simulink model "Essaie_01"  (R2021a)
settings: Solver=FixedStepDiscrete  StartTime=0.0  StopTime=8.75  RelTol=1e-3  EnableMultiTasking=on
libraries: simulink x8, simulink_extras x2, dspsigops x2, dsparch4 x2, commfilt2 x2
settings Model: Creator=sebastienroy  LastModifiedBy=Simon
settings SolverCC: AlgebraicLoopSolver=TrustRegion
settings DataIOCC: LimitDataPoints=on  SaveFormat=Array  ReturnWorkspaceOutputs=off
settings OptimizationCC: LifeSpan=inf
settings DebuggingCC: UnderspecifiedInitializationDetection=Classic  MergeDetectMultiDrivingBlocksExec=none  SolverPrmCheckMsg=warning  StateNameClashWarn=warning  SFUnexpectedBacktrackingDiag=warning  SFNoUnconditionalDefaultTransitionDiag=warning  SFExecutionAtInitializationDiag=none  SFMachineParentedDataDiag=warning  ArithmeticOperatorsInVariantConditions=warning
settings HardwareCC: ProdBitPerPointer=32  ProdBitPerSizeT=32  ProdBitPerPtrDiffT=32  ProdLargestAtomicFloat=None  ProdIntDivRoundTo=Undefined  ProdEndianess=Unspecified  ProdWordSize=32  ProdHWDeviceType=32-bit Generic
settings ModelReferenceCC: PropagateSignalLabelsOutOfModel=off
settings SFSimCC: SimUseLocalCustomCode=off  CustomCodeUndefinedFunction=UseInterfaceOnly
settings RTWCC: RTWUseLocalCustomCode=off
settings CodeAppCC: StateflowObjectComments=on
settings GRTTargetCC: TargetLangStandard=C89/C90 (ANSI)
settings ConfigComp: CovMetricSettings=dw  CovSaveCumulativeToWorkspaceVar=on  CovSaveSingleToWorkspaceVar=on  CovExternalEMLEnable=off

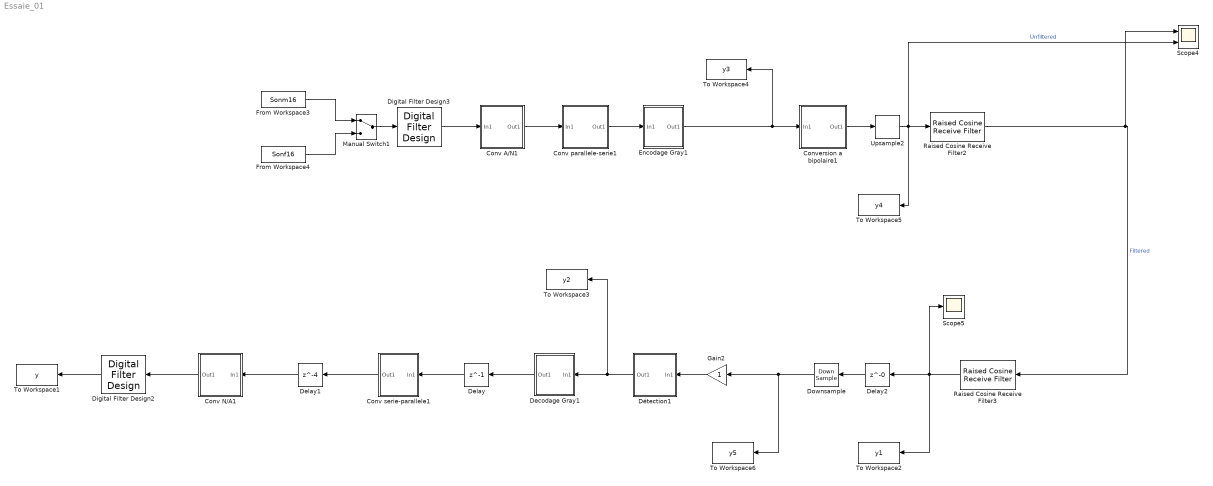
== system Essaie_01 ==
  Conv A/N1 : Subsystem
  Conv N/A1 : Subsystem
  Conv parallele-serie1 : Subsystem
  Conv serie-parallele1 : Subsystem
  Conversion a bipolaire1 : Subsystem
  Decodage Gray1 : Subsystem
  Delay : Delay  DelayLength=1  InitialCondition=0
  Delay1 : Delay  DelayLength=4  InitialCondition=0
  Delay2 : Delay  DelayLength=0  InitialCondition=0
  Digital Filter Design2 : dsparch4/Digital Filter Design  mwdsp_browser_bugfix_var=off
  Digital Filter Design3 : dsparch4/Digital Filter Design  mwdsp_browser_bugfix_var=off
  Downsample : DownSample  N=20  RateOptions=Allow multirate processing
  Détection1 : Subsystem
  Encodage Gray1 : Subsystem
  From Workspace3 : FromWorkspace  VariableName=Sonm16  SampleTime=1/16000  Interpolate=off  OutputAfterFinalValue=Setting to zero
  From Workspace4 : FromWorkspace  VariableName=Sonf16  SampleTime=1/16000  Interpolate=off  OutputAfterFinalValue=Setting to zero
  Gain2 : Gain
  Manual Switch1 : ManualSwitch
  Raised Cosine Receive Filter2 : commfilt2/Raised Cosine Receive Filter  filtType=Square root  R=0.2  filtSpan=10  N=20  downFactor=1  downOffset=0  filterGain=1  RateOptions=Allow multirate processing  framing=Mute  checkCoeff=on  variableName=rcRxFilt2  currentFiltSpan=10  D=5  inputOffset=0  sampMode=Mute  saveAsFlag=0  rateMode=Downsampling  checkGain=Normalized  launchFVT=on  roundingMode=Floor  overflowMode=off  coeffDataTypeStr=Inherit: Same word length as input  coeffMin=[]  coeffMax=[]  coeffLastDataTypeStr=Inherit: Same word length as input  accumDataTypeStr=Inherit: Same as product output  accumLastDataTypeStr=Inherit: Same as product output  outputDataTypeStr=Inherit: Same as accumulator  outputMin=[]  outputMax=[]  outputLastDataTypeStr=Inherit: Same as accumulator
  Raised Cosine Receive Filter3 : commfilt2/Raised Cosine Receive Filter  filtType=Square root  R=0.2  filtSpan=10  N=20  downFactor=1  downOffset=0  filterGain=1  RateOptions=Allow multirate processing  framing=Mute  checkCoeff=on  variableName=rcRxFilt3  currentFiltSpan=10  D=5  inputOffset=0  sampMode=Mute  saveAsFlag=0  rateMode=Downsampling  checkGain=Normalized  launchFVT=on  roundingMode=Floor  overflowMode=off  coeffDataTypeStr=Inherit: Same word length as input  coeffMin=[]  coeffMax=[]  coeffLastDataTypeStr=Inherit: Same word length as input  accumDataTypeStr=Inherit: Same as product output  accumLastDataTypeStr=Inherit: Same as product output  outputDataTypeStr=Inherit: Same as accumulator  outputMin=[]  outputMax=[]  outputLastDataTypeStr=Inherit: Same as accumulator
  Scope4 : Scope  NumInputPorts=2
  Scope5 : Scope
  To Workspace1 : ToWorkspace  VariableName=y  SampleTime=-1
      settings: Save2DSignal=2-D array (concatenate along first dimension)
  To Workspace2 : ToWorkspace  VariableName=y1  SampleTime=-1
      settings: Save2DSignal=2-D array (concatenate along first dimension)
  To Workspace3 : ToWorkspace  VariableName=y2  SampleTime=-1
      settings: Save2DSignal=2-D array (concatenate along first dimension)
  To Workspace4 : ToWorkspace  VariableName=y3  SampleTime=-1
      settings: Save2DSignal=2-D array (concatenate along first dimension)
  To Workspace5 : ToWorkspace  VariableName=y4  SampleTime=-1
      settings: Save2DSignal=2-D array (concatenate along first dimension)
  To Workspace6 : ToWorkspace  VariableName=y5  SampleTime=-1
      settings: Save2DSignal=2-D array (concatenate along first dimension)
  Upsample2 : dspsigops/Upsample  N=20  phase=0  RateOptions=Allow multirate processing  ic=0  mode=Unused parameter value
  wires:
  Upsample2/1 -> Scope4/2, Raised Cosine Receive Filter2/1, To Workspace5/1  "Unfiltered"
  Encodage Gray1/1(Out1) -> To Workspace4/1, Conversion a bipolaire1/1(In1)
  Conv A/N1/1(Out1) -> Conv parallele-serie1/1(In1)
  Decodage Gray1/1(Out1) -> Delay/1
  Digital Filter Design3/1 -> Conv A/N1/1(In1)
  Gain2/1 -> Détection1/1(In1)
  Delay2/1 -> Downsample/1
  Conv N/A1/1(Out1) -> Digital Filter Design2/1
  From Workspace3/1 -> Manual Switch1/1
  Détection1/1(Out1) -> To Workspace3/1, Decodage Gray1/1(In1)
  Conversion a bipolaire1/1(Out1) -> Upsample2/1
  Conv parallele-serie1/1(Out1) -> Encodage Gray1/1(In1)
  Manual Switch1/1 -> Digital Filter Design3/1
  Downsample/1 -> To Workspace6/1, Gain2/1
  Delay/1 -> Conv serie-parallele1/1(In1)
  Raised Cosine Receive Filter2/1 -> Raised Cosine Receive Filter3/1, Scope4/1  "Filtered"
  Digital Filter Design2/1 -> To Workspace1/1
  From Workspace4/1 -> Manual Switch1/2
  Raised Cosine Receive Filter3/1 -> Scope5/1, To Workspace2/1, Delay2/1
  Delay1/1 -> Conv N/A1/1(In1)
  Conv serie-parallele1/1(Out1) -> Delay1/1

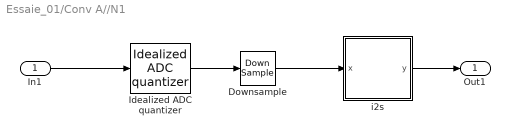
== system Essaie_01/Conv A//N1 ==
  In1 : Inport
  Downsample : DownSample  RateOptions=Allow multirate processing
  Idealized ADC quantizer : simulink_extras/Additional Discrete/Idealized ADC quantizer  NumberOfConverterBits=8  Vmin=-1  Vmax=1  OutputDataType=double  OutputNegativeValues=off
  i2s : Subsystem
  Out1 : Outport  VectorParamsAs1DForOutWhenUnconnected=off
  wires:
  Idealized ADC quantizer/1 -> Downsample/1
  In1/1 -> Idealized ADC quantizer/1
  Downsample/1 -> i2s/1(x)
  i2s/1(y) -> Out1/1

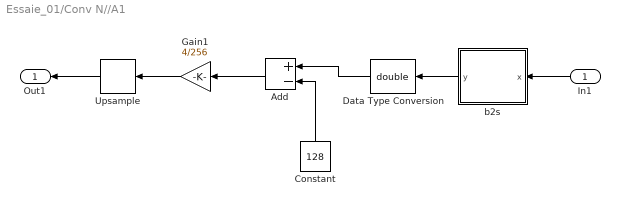
== system Essaie_01/Conv N//A1 ==
  In1 : Inport
  Add : Sum  Inputs=+-
  Constant : Constant  Value=128
  Data Type Conversion : DataTypeConversion  OutDataTypeStr=double
  Gain1 : Gain  Gain=4/256
  Upsample : dspsigops/Upsample  N=2  phase=0  RateOptions=Allow multirate processing  ic=0  mode=Unused parameter value
  b2s : Subsystem
  Out1 : Outport  VectorParamsAs1DForOutWhenUnconnected=off
  wires:
  Upsample/1 -> Out1/1
  Gain1/1 -> Upsample/1
  Constant/1 -> Add/2
  Data Type Conversion/1 -> Add/1
  Add/1 -> Gain1/1
  In1/1 -> b2s/1(x)
  b2s/1(y) -> Data Type Conversion/1

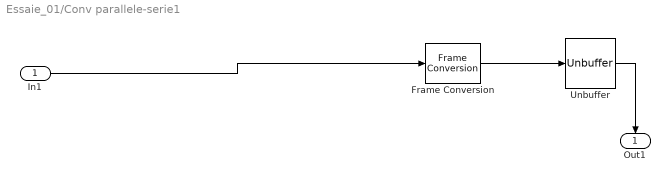
== system Essaie_01/Conv parallele-serie1 ==
  In1 : Inport
  Frame Conversion : FrameConversion
  Unbuffer : Unbuffer
  Out1 : Outport  VectorParamsAs1DForOutWhenUnconnected=off
  wires:
  Frame Conversion/1 -> Unbuffer/1
  Unbuffer/1 -> Out1/1
  In1/1 -> Frame Conversion/1

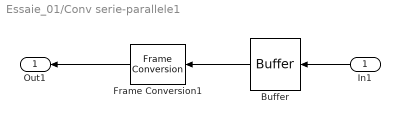
== system Essaie_01/Conv serie-parallele1 ==
  In1 : Inport
  Buffer : Buffer  N=4
  Frame Conversion1 : FrameConversion  OutFrame=Sample-based
  Out1 : Outport  VectorParamsAs1DForOutWhenUnconnected=off
  wires:
  Frame Conversion1/1 -> Out1/1
  In1/1 -> Buffer/1
  Buffer/1 -> Frame Conversion1/1

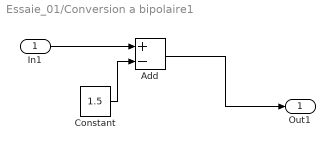
== system Essaie_01/Conversion a bipolaire1 ==
  In1 : Inport
  Add : Sum  Inputs=+-
  Constant : Constant  Value=1.5
  Out1 : Outport  VectorParamsAs1DForOutWhenUnconnected=off
  wires:
  In1/1 -> Add/1
  Add/1 -> Out1/1
  Constant/1 -> Add/2

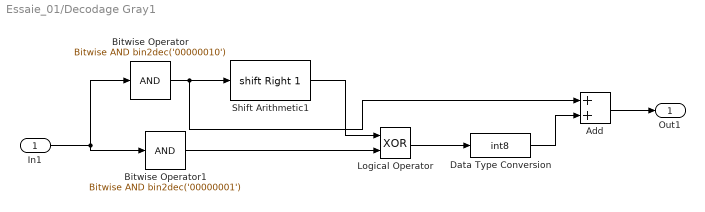
== system Essaie_01/Decodage Gray1 ==
  In1 : Inport
  Add : Sum
  Bitwise Operator : simulink/Logic and Bit Operations/Bitwise Operator  logicop=AND  UseBitMask=on  BitMask=bin2dec('00000010')  BitMaskRealWorld=Stored Integer
  Bitwise Operator1 : simulink/Logic and Bit Operations/Bitwise Operator  logicop=AND  UseBitMask=on  BitMask=bin2dec('00000001')  BitMaskRealWorld=Stored Integer
  Data Type Conversion : DataTypeConversion  OutDataTypeStr=int8
  Logical Operator : Logic  Operator=XOR  AllPortsSameDT=off
  Shift Arithmetic1 : ArithShift  BitShiftNumber=1  BitShiftDirection=Right
  Out1 : Outport  VectorParamsAs1DForOutWhenUnconnected=off
  wires:
  In1/1 -> Bitwise Operator/1, Bitwise Operator1/1
  Bitwise Operator/1 -> Add/1, Shift Arithmetic1/1
  Shift Arithmetic1/1 -> Logical Operator/1
  Bitwise Operator1/1 -> Logical Operator/2
  Add/1 -> Out1/1
  Logical Operator/1 -> Data Type Conversion/1
  Data Type Conversion/1 -> Add/2

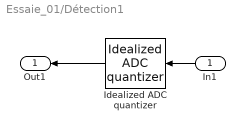
== system Essaie_01/Détection1 ==
  In1 : Inport
  Idealized ADC quantizer : simulink_extras/Additional Discrete/Idealized ADC quantizer  NumberOfConverterBits=2  Vmin=-1.5*20  Vmax=2.5*20  OutputDataType=int8  OutputNegativeValues=off
  Out1 : Outport
  wires:
  In1/1 -> Idealized ADC quantizer/1
  Idealized ADC quantizer/1 -> Out1/1

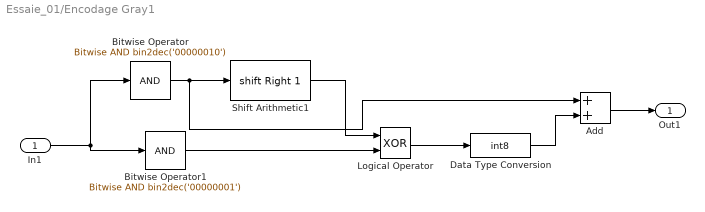
== system Essaie_01/Encodage Gray1 ==
  In1 : Inport
  Add : Sum
  Bitwise Operator : simulink/Logic and Bit Operations/Bitwise Operator  logicop=AND  UseBitMask=on  BitMask=bin2dec('00000010')  BitMaskRealWorld=Stored Integer
  Bitwise Operator1 : simulink/Logic and Bit Operations/Bitwise Operator  logicop=AND  UseBitMask=on  BitMask=bin2dec('00000001')  BitMaskRealWorld=Stored Integer
  Data Type Conversion : DataTypeConversion  OutDataTypeStr=int8
  Logical Operator : Logic  Operator=XOR  AllPortsSameDT=off
  Shift Arithmetic1 : ArithShift  BitShiftNumber=1  BitShiftDirection=Right
  Out1 : Outport  VectorParamsAs1DForOutWhenUnconnected=off
  wires:
  In1/1 -> Bitwise Operator/1, Bitwise Operator1/1
  Bitwise Operator/1 -> Add/1, Shift Arithmetic1/1
  Shift Arithmetic1/1 -> Logical Operator/1
  Bitwise Operator1/1 -> Logical Operator/2
  Add/1 -> Out1/1
  Logical Operator/1 -> Data Type Conversion/1
  Data Type Conversion/1 -> Add/2

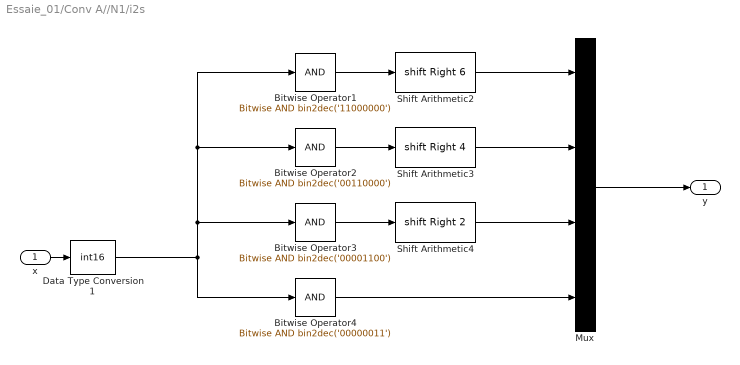
== system Essaie_01/Conv A//N1/i2s ==
  x : Inport
  Bitwise Operator1 : simulink/Logic and Bit Operations/Bitwise Operator  logicop=AND  UseBitMask=on  BitMask=bin2dec('11000000')  BitMaskRealWorld=Stored Integer
  Bitwise Operator2 : simulink/Logic and Bit Operations/Bitwise Operator  logicop=AND  UseBitMask=on  BitMask=bin2dec('00110000')  BitMaskRealWorld=Stored Integer
  Bitwise Operator3 : simulink/Logic and Bit Operations/Bitwise Operator  logicop=AND  UseBitMask=on  BitMask=bin2dec('00001100')  BitMaskRealWorld=Stored Integer
  Bitwise Operator4 : simulink/Logic and Bit Operations/Bitwise Operator  logicop=AND  UseBitMask=on  BitMask=bin2dec('00000011')  BitMaskRealWorld=Stored Integer
  Data Type Conversion1 : DataTypeConversion  OutDataTypeStr=int16
  Mux : Mux
  Shift Arithmetic2 : ArithShift  BitShiftNumber=6  BitShiftDirection=Right
  Shift Arithmetic3 : ArithShift  BitShiftNumber=4  BitShiftDirection=Right
  Shift Arithmetic4 : ArithShift  BitShiftNumber=2  BitShiftDirection=Right
  y : Outport  VectorParamsAs1DForOutWhenUnconnected=off
  wires:
  x/1 -> Data Type Conversion1/1
  Data Type Conversion1/1 -> Bitwise Operator2/1, Bitwise Operator1/1, Bitwise Operator3/1, Bitwise Operator4/1
  Bitwise Operator1/1 -> Shift Arithmetic2/1
  Bitwise Operator2/1 -> Shift Arithmetic3/1
  Bitwise Operator3/1 -> Shift Arithmetic4/1
  Bitwise Operator4/1 -> Mux/4
  Mux/1 -> y/1
  Shift Arithmetic3/1 -> Mux/2
  Shift Arithmetic4/1 -> Mux/3
  Shift Arithmetic2/1 -> Mux/1

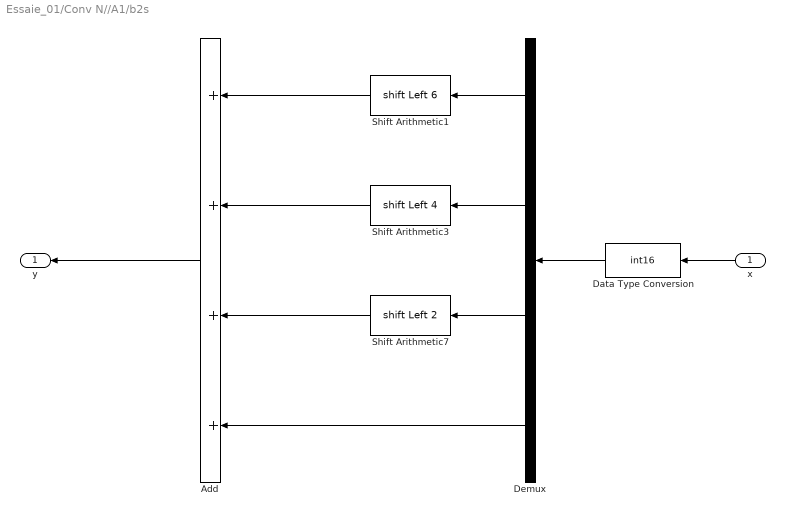
== system Essaie_01/Conv N//A1/b2s ==
  x : Inport
  Add : Sum  Inputs=++++
  Data Type Conversion : DataTypeConversion  OutDataTypeStr=int16  RndMeth=Round
  Demux : Demux
  Shift Arithmetic1 : ArithShift  BitShiftNumber=6  BitShiftDirection=Left
  Shift Arithmetic3 : ArithShift  BitShiftNumber=4  BitShiftDirection=Left
  Shift Arithmetic7 : ArithShift  BitShiftNumber=2  BitShiftDirection=Left
  y : Outport  VectorParamsAs1DForOutWhenUnconnected=off
  wires:
  Demux/4 -> Add/4
  Shift Arithmetic7/1 -> Add/3
  Shift Arithmetic3/1 -> Add/2
  Shift Arithmetic1/1 -> Add/1
  Demux/2 -> Shift Arithmetic3/1
  Demux/3 -> Shift Arithmetic7/1
  Demux/1 -> Shift Arithmetic1/1
  Data Type Conversion/1 -> Demux/1
  Add/1 -> y/1
  x/1 -> Data Type Conversion/1
